simulink model "encoder_easy_example"  (R2018b)
settings: Solver=FixedStepAuto  StartTime=0.0  StopTime=inf  RelTol=1e-3  EnableMultiTasking=on
undefined symbols (not defined in the file): ee_sli_rtmsupport, gcbh
libraries: simulink x3, mbedblockslib x2
settings Model: SimulationMode=accelerator  ExtModeTrigDuration=10  Creator=pokpong.c  LastModifiedBy=szgno
settings SolverCC: PositivePriorityOrder=on
settings DataIOCC: ReturnWorkspaceOutputs=on
settings OptimizationCC: StrengthReduction=on  PassReuseOutputArgsAs=Individual arguments  ZeroExternalMemoryAtStartup=off  ZeroInternalMemoryAtStartup=off  MaxStackSize=64  OptimizeBlockOrder=speed  OptimizationPriority=Speed  OptimizationCustomize=off
settings DebuggingCC: ParameterTunabilityLossMsg=error
settings HardwareCC: ProdBitPerPointer=32  ProdBitPerSizeT=32  ProdBitPerPtrDiffT=32  ProdLargestAtomicInteger=Long  ProdLargestAtomicFloat=Double  ProdWordSize=32  ProdHWDeviceType=ARM Compatible->ARM Cortex
settings ModelReferenceCC: ModelReferenceNumInstancesAllowed=Single
settings SFSimCC: MATLABDynamicMemAlloc=off
settings RTWCC: SystemTargetFile=ert.tlc  HardwareBoard=STM32 Nucleo F411RE  TemplateMakefile=ert_default_tmf  GenerateReport=on  Toolchain=GNU Tools for ARM Embedded Processors  IncludeHyperlinkInReport=on  LaunchReport=on  GenerateTraceInfo=on  GenerateTraceReport=on  GenerateTraceReportSl=on  GenerateTraceReportSf=on  GenerateTraceReportEml=on
settings CodeAppCC: ForceParamTrailComments=on  IgnoreCustomStorageClasses=off  OperatorAnnotations=on  SimulinkDataObjDesc=on  SFDataObjDesc=on  InsertBlockDesc=on
settings ERTTargetCC: SupportContinuousTime=on  ExtModeStaticAllocSize=2000

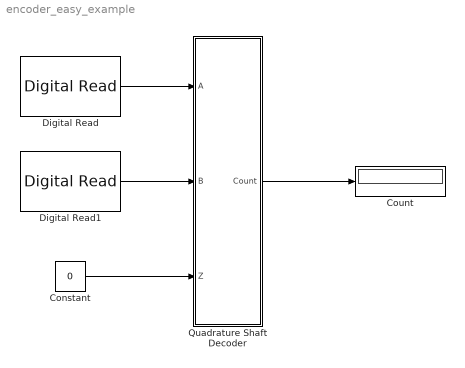
== system encoder_easy_example ==
  Constant : Constant  Value=0
  Count : Display
  Digital Read : mbedblockslib/Digital Read  Pin=PC_0  Direction=input  SampleTime=0.001
      settings: SourceProductBaseCode=MICROBIT,NUCLEO,STMICRODIS
  Digital Read1 : mbedblockslib/Digital Read  Pin=PC_1  Direction=input  SampleTime=0.001
      settings: SourceProductBaseCode=MICROBIT,NUCLEO,STMICRODIS
  Quadrature Shaft Decoder : Subsystem  AncestorBlock=eeQuadratureDecoder/Quadrature Shaft Decoder  LoadFcn=ee_sli_rtmsupport( 'loadfcn', gcbh );  mask(Quadrature Shaft Decoder){NPulse=1, Ts=0.001}
      mask prompts: NPulse "physmod:ee:library:comments:control:eeQuadratureDecoder:PulsesPerRevolutio_MP"; Ts "physmod:ee:library:comments:control:eeQuadratureDecoder:SampleTime1ForInherited_MP"
      mask help: physmod:ee:library:comments:control:eeQuadratureDecoder:QuadratureDecoder_MD
      mask init:
      | if Ts <= 0 && Ts ~= -1            
      |     error(message('physmod:ee:library:MinusOneOrPositive',getString(message('physmod:ee:library:comments:control:eeResolverToDigitalConverter:SampleTime1ForInherited_MP'))));            
      | end
      | 
      | if NPulse <= 0          
      |     error(message('physmod:simscape:compiler:patterns:checks:GreaterThanZero',getString(message('physmod:ee:library:comments:control:eeQuadratureDecoder:PulsesPerRevolutio_MP'))));            
      | end
      settings: CopyFcn=ee_sli_rtmsupport( 'copyfcn', gcbh );  DeleteFcn=ee_sli_rtmsupport( 'deletefcn', gcbh );  ModelCloseFcn=ee_sli_rtmsupport( 'modelclosefcn', gcbh );  PostSaveFcn=ee_sli_rtmsupport( 'postsavefcn', gcbh );  PreCopyFcn=ee_sli_rtmsupport( 'precopyfcn', gcbh );  OpenFcn=ee_sli_rtmsupport( 'openfcn', gcbh );  CloseFcn=ee_sli_rtmsupport( 'closefcn', gcbh );  PreDeleteFcn=ee_sli_rtmsupport( 'predeletefcn', gcbh );
      mask Help: web(nesl_help(gcbh))
      mask DialogControl NPulse Prompt: Pulses per revolution
      mask DialogControl Ts Prompt: Sample time (-1 for inherited)
  wires:
  Digital Read1/1 -> Quadrature Shaft Decoder/2(B)
  Digital Read/1 -> Quadrature Shaft Decoder/1(A)
  Constant/1 -> Quadrature Shaft Decoder/3(Z)
  Quadrature Shaft Decoder/1(Count) -> Count/1

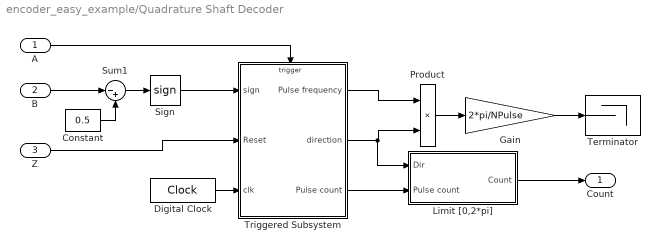
== system encoder_easy_example/Quadrature Shaft Decoder ==
  A : Inport  SampleTime=Ts
  B : Inport  Port=2  SampleTime=Ts
  Z : Inport  Port=3  SampleTime=Ts
  Constant : Constant  Value=0.5  SampleTime=Ts
  Digital Clock : DigitalClock  SampleTime=Ts
  Gain : Gain  Gain=2*pi/NPulse
  Limit [0,2*pi] : Subsystem
  Product : Product
  Sign : Signum
  Sum1 : Sum  Inputs=|-+
  Terminator : Terminator
  Triggered Subsystem : Subsystem  TreatAsAtomicUnit=on
  Count : Outport  VectorParamsAs1DForOutWhenUnconnected=off
  wires:
  Digital Clock/1 -> Triggered Subsystem/3(clk)
  Sign/1 -> Triggered Subsystem/1(sign)
  A/1 -> Triggered Subsystem/Trigger
  B/1 -> Sum1/1
  Sum1/1 -> Sign/1
  Constant/1 -> Sum1/2
  Triggered Subsystem/1(Pulse frequency) -> Product/1
  Triggered Subsystem/2(direction) -> Limit [0,2*pi]/1(Dir), Product/2
  Product/1 -> Gain/1
  Gain/1 -> Terminator/1
  Z/1 -> Triggered Subsystem/2(Reset)
  Triggered Subsystem/3(Pulse count) -> Limit [0,2*pi]/2(Pulse count)
  Limit [0,2*pi]/1(Count) -> Count/1

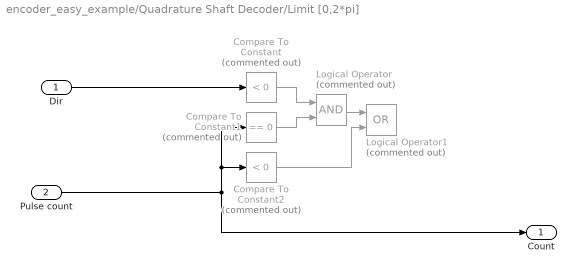
== system encoder_easy_example/Quadrature Shaft Decoder/Limit [0,2*pi] ==
  Dir : Inport
  Pulse count : Inport  Port=2
  Compare To Constant : simulink/Logic and Bit Operations/Compare To Constant  Commented=on  relop=<  const=0  OutDataTypeStr=boolean
  Compare To Constant1 : simulink/Logic and Bit Operations/Compare To Constant  Commented=on  relop===  const=0  OutDataTypeStr=boolean
  Compare To Constant2 : simulink/Logic and Bit Operations/Compare To Constant  Commented=on  relop=<  const=0  OutDataTypeStr=boolean
  Logical Operator : Logic  Commented=on  AllPortsSameDT=off  OutDataTypeStr=boolean
  Logical Operator1 : Logic  Commented=on  Operator=OR  AllPortsSameDT=off  OutDataTypeStr=boolean
  Count : Outport  VectorParamsAs1DForOutWhenUnconnected=off
  wires:
  Dir/1 -> Compare To Constant/1
  Compare To Constant/1 -> Logical Operator/1
  Compare To Constant1/1 -> Logical Operator/2
  Logical Operator/1 -> Logical Operator1/1
  Pulse count/1 -> Count/1, Compare To Constant2/1, Compare To Constant1/1
  Compare To Constant2/1 -> Logical Operator1/2

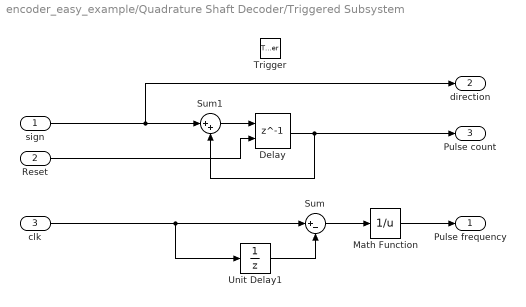
== system encoder_easy_example/Quadrature Shaft Decoder/Triggered Subsystem ==
  sign : Inport
  Reset : Inport  Port=2
  clk : Inport  Port=3
  Trigger : TriggerPort  VariantControl=Variant
  Delay : Delay  DelayLength=1  InitialCondition=0  ExternalReset=Rising
      settings: InputPortMap=u0,r5
  Math Function : Math  Operator=reciprocal  SaturateOnIntegerOverflow=on
  Sum : Sum  Inputs=|+-
  Sum1 : Sum  Inputs=|++
  Unit Delay1 : UnitDelay  InitialCondition=-1e10  SampleTime=-1  HasFrameUpgradeWarning=on
  Pulse frequency : Outport  VectorParamsAs1DForOutWhenUnconnected=off
  direction : Outport  Port=2  InitialOutput=0  VectorParamsAs1DForOutWhenUnconnected=off
  Pulse count : Outport  Port=3  InitialOutput=0  VectorParamsAs1DForOutWhenUnconnected=off
  wires:
  Sum1/1 -> Delay/1
  sign/1 -> Sum1/1, direction/1
  Delay/1 -> Pulse count/1, Sum1/2
  clk/1 -> Unit Delay1/1, Sum/1
  Unit Delay1/1 -> Sum/2
  Sum/1 -> Math Function/1
  Math Function/1 -> Pulse frequency/1
  Reset/1 -> Delay/2
